simulink model "VAJA3_1"  (R2020a)
settings: Solver=VariableStepAuto  StartTime=0.0  StopTime=15000  RelTol=1e-3
undefined symbols (not defined in the file): a, b
settings Model: Creator=Jaka  LastModifiedBy=Jaka

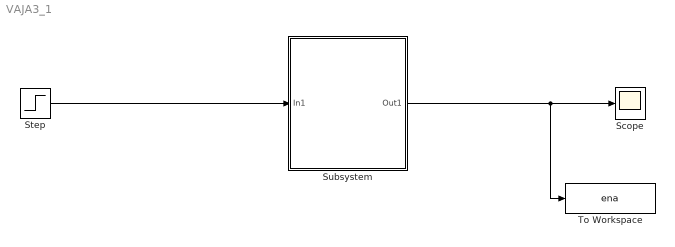
== system VAJA3_1 ==
  Scope : Scope
  Step : Step  SampleTime=0
  Subsystem : Subsystem
  To Workspace : ToWorkspace  VariableName=ena  SampleTime=-1
  wires:
  Subsystem/1(Out1) -> To Workspace/1, Scope/1
  Step/1 -> Subsystem/1(In1)

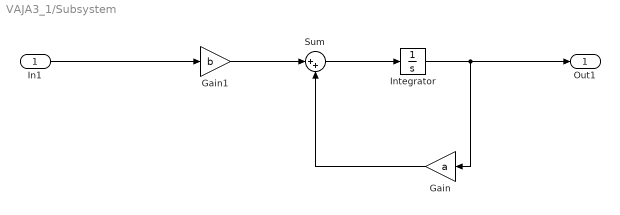
== system VAJA3_1/Subsystem ==
  In1 : Inport
  Gain : Gain  Gain=a
  Gain1 : Gain  Gain=b
  Integrator : Integrator  InitialCondition=-5
  Sum : Sum  Inputs=|++
  Out1 : Outport
  wires:
  Gain/1 -> Sum/2
  In1/1 -> Gain1/1
  Integrator/1 -> Out1/1, Gain/1
  Gain1/1 -> Sum/1
  Sum/1 -> Integrator/1
